simulink model "system_model"  (R2013b)
settings: Solver=ode3  SolverMode=MultiTasking  StartTime=0.0  StopTime=10.0  FixedStep=0.01  RelTol=1e-3
libraries: simulink x3, sw_lib x1
settings Model: ExtModeTrigDuration=2  Creator=raarenst  LastModifiedBy=raarenst
settings SolverCC: AutoInsertRateTranBlk=on
settings DataIOCC: SignalLoggingSaveFormat=ModelDataLogs
settings OptimizationCC: OptimizeModelRefInitCode=on  LifeSpan=1
settings DebuggingCC: UnderspecifiedInitializationDetection=Simplified  SolverPrmCheckMsg=none  MultiTaskDSMMsg=warning  MultiTaskCondExecSysMsg=none  ParameterPrecisionLossMsg=none  StrictBusMsg=None
settings HardwareCC: ProdBitPerInt=16  ProdBitPerPointer=8  ProdIntDivRoundTo=Zero  ProdEndianess=LittleEndian  ProdWordSize=8  ProdHWDeviceType=Atmel->AVR
settings RTWCC: SystemTargetFile=realtime.tlc  GenerateMakefile=off  TemplateMakefile=realtime.tmf  Description=Run on Target Hardware  RTWVerbose=off  ProcessScript=realtime_make_rtw_hook  IncludeERTFirstTime=on
settings STFCustomTargetCC: TargetLibSuffix=.a  CodeReplacementLibrary=None  GenerateSampleERTMain=on  ERTCustomFileBanners=on  SupportNonInlinedSFcns=off  SupportVariableSizeSignals=on  MATLABClassNameForMDSCustomization=Simulink.SoftwareTarget.ERTCustomization  GRTInterface=off  SystemTargetFile=realtime.tlc
settings ERTTargetCC: GenerateSampleERTMain=on  ParMdlRefBuildCompliant=off  CompOptLevelCompliant=off  ConcurrentExecutionCompliant=off  CombineOutputUpdateFcns=off  ERTFirstTimeCompliant=off  SupportContinuousTime=on  SupportVariableSizeSignals=on  ModelStepFunctionPrototypeControlCompliant=off  CPPClassGenCompliant=off  ExtModeTransport=3  ExtModeMexFile=ext_serial_win32_comm  ExtModeMexArgs=0 1 9600  InlinedParameterPlacement=NonHierarchical  ERTSrcFileBannerTemplate=realtime_code_template.cgt  ERTHdrFileBannerTemplate=realtime_code_template.cgt  ERTDataSrcFileTemplate=realtime_code_template.cgt  ERTDataHdrFileTemplate=realtime_code_template.cgt  ERTCustomFileTemplate=realtime_file_process.tlc
settings ConfigurationSet: Description=SimMechanics 2G

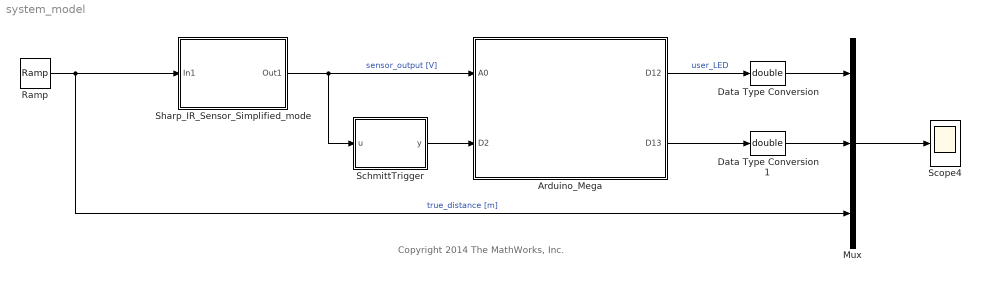
== system system_model ==
  note: Copyright 2014 The MathWorks, Inc.
  Arduino_Mega : Subsystem
      mask Display:
      | image('arduino_mega.jpg');
      | port_label('input', 1, 'A0');
      | port_label('input', 2, 'D2');
      | port_label('output', 1, 'D12');
      | port_label('output', 2, 'D13');
  Data Type Conversion : DataTypeConversion  OutDataTypeStr=double
  Data Type Conversion1 : DataTypeConversion  OutDataTypeStr=double
  Mux : Mux  Inputs=3
  Ramp : simulink/Sources/Ramp  slope=-0.1  start=0  X0=1
  SchmittTrigger : MATLAB Function  TreatAsAtomicUnit=on
  Scope4 : Scope
      settings: YMin=0.2  YMax=1  SaveName=ScopeData4
  Sharp_IR_Sensor_Simplified_mode : Subsystem
      mask Display: image('sharp_ir.jpg');
  wires:
  Ramp/1 -> Mux/3, Sharp_IR_Sensor_Simplified_mode/1(In1)  "true_distance [m]"
  Sharp_IR_Sensor_Simplified_mode/1(Out1) -> SchmittTrigger/1(u), Arduino_Mega/1(A0)  "sensor_output [V]"
  Arduino_Mega/1(D12) -> Data Type Conversion/1  "user_LED"
  Data Type Conversion/1 -> Mux/1
  Mux/1 -> Scope4/1
  Arduino_Mega/2(D13) -> Data Type Conversion1/1
  Data Type Conversion1/1 -> Mux/2
  SchmittTrigger/1(y) -> Arduino_Mega/2(D2)

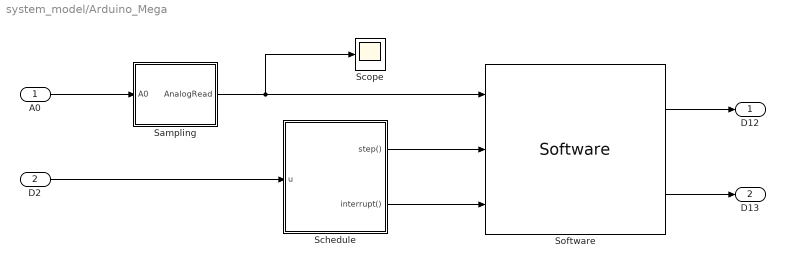
== system system_model/Arduino_Mega ==
  A0 : Inport
  D2 : Inport  Port=2
  Sampling : Subsystem
  Schedule : MATLAB Function  TreatAsAtomicUnit=on
  Scope : Scope
  Software : sw_lib/Software
  D12 : Outport
  D13 : Outport  Port=2
  wires:
  Software/1 -> D12/1
  A0/1 -> Sampling/1(A0)
  Sampling/1(AnalogRead) -> Software/1, Scope/1
  Software/2 -> D13/1
  D2/1 -> Schedule/1(u)
  Schedule/2(interrupt()) -> Software/3
  Schedule/1(step()) -> Software/2

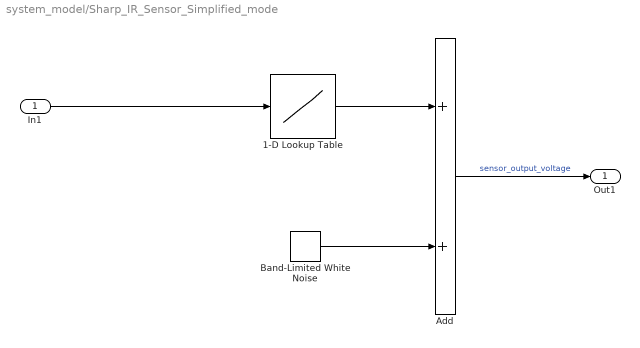
== system system_model/Sharp_IR_Sensor_Simplified_mode ==
  In1 : Inport
  1-D Lookup Table : Lookup_n-D  NumberOfTableDimensions=1  BreakpointsForDimension1="[0 10   15     20 30 40    50  60   70  80  90 100 110 120 130 140 150 ]/100"  Table="[0 2.3 2.75 2.55 2 1.55 1.25 1.05 0.9 0.8 0.725 0.65 0.6 0.55  0.5 0.495 0.49 ]"  InternalRulePriority=Speed  RndMeth=Simplest  InputSameDT=on
  Add : Sum
  Band-Limited White Noise : simulink/Sources/Band-Limited White Noise  Cov=[0.0000000001]  Ts=0.01  seed=[23341]
  Out1 : Outport
  wires:
  Band-Limited White Noise/1 -> Add/2
  1-D Lookup Table/1 -> Add/1
  In1/1 -> 1-D Lookup Table/1
  Add/1 -> Out1/1  "sensor_output_voltage"

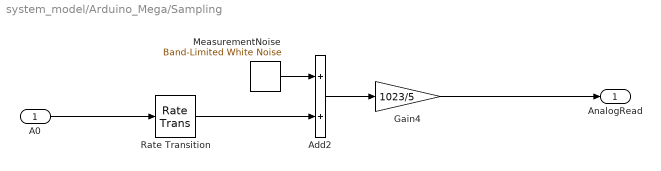
== system system_model/Arduino_Mega/Sampling ==
  A0 : Inport
  Add2 : Sum
  Gain4 : Gain  Gain=1023/5  OutDataTypeStr=uint16  SaturateOnIntegerOverflow=on
  MeasurementNoise : simulink/Sources/Band-Limited White Noise  Cov=[0.000001]  Ts=0.1  seed=[2334]
  Rate Transition : RateTransition  OutPortSampleTime=0.1
  AnalogRead : Outport
  wires:
  Gain4/1 -> AnalogRead/1
  A0/1 -> Rate Transition/1
  Add2/1 -> Gain4/1
  Rate Transition/1 -> Add2/2
  MeasurementNoise/1 -> Add2/1

== matlab function system_model/Arduino_Mega/Schedule ==
  settings: updateMethod=DISCRETE  sampleTime=0.01
  data: u input
  events: step output FUNCTION_CALL_EVENT; interrupt output FUNCTION_CALL_EVENT
function fcn(u)
%#codegen

persistent counter;
persistent state;
state_low = 0;
state_high = 1;

if isempty(state)
   state = state_low;
   counter = 0;
end

if counter == 10
   step();
   counter = 0;
else
    counter = counter + 1;
end

if state == state_low
    if u > 2.5
        state = state_high;
        interrupt();
    end
else
    if u <= 2.5
        state = state_low;
        interrupt();
    end
end

== matlab function system_model/SchmittTrigger ==
  settings: updateMethod=DISCRETE  sampleTime=0.01
  data: u input; y output
function y = fcn(u)
%#codegen

state_low = 0;
state_high = 1;
persistent state;

threshold_low = 2.0;
threshold_high = 2.3;

output_low = 1.3;
output_high = 4.7;

if isempty(state)
    % Initial value
    state = state_low;
end

if state == state_low
     if (u < threshold_high)
         y = output_low;
     else
        y = output_high;
        state = state_high;
     end
else          
    if (u > threshold_low)
        y = output_high;
    else
        y = output_low;
        state = state_low;
    end
end
